simulink model "template_2018a"  (R2018a)
settings: Solver=ode45  StartTime=0.0  StopTime=0.75  MaxStep=1e-4  RelTol=1e-3  EnableMultiTasking=on
undefined symbols (not defined in the file or in its folder): KD, KI, KP
settings Model: Creator=Joe  LastModifiedBy=Adam Minnich
settings DataIOCC: LimitDataPoints=on  SaveFormat=Array
settings OptimizationCC: LifeSpan=inf
settings DebuggingCC: UnderspecifiedInitializationDetection=Classic  MergeDetectMultiDrivingBlocksExec=none  SolverPrmCheckMsg=warning  SFUnexpectedBacktrackingDiag=warning  SFNoUnconditionalDefaultTransitionDiag=warning  SFExecutionAtInitializationDiag=none
settings HardwareCC: ProdBitPerPointer=32  ProdBitPerSizeT=32  ProdBitPerPtrDiffT=32  ProdLargestAtomicFloat=None  ProdIntDivRoundTo=Undefined  ProdEndianess=Unspecified  ProdWordSize=32  ProdHWDeviceType=32-bit Generic
settings ModelReferenceCC: PropagateSignalLabelsOutOfModel=off
settings CodeAppCC: StateflowObjectComments=on
settings GRTTargetCC: TargetLangStandard=C89/C90 (ANSI)  GeneratePreprocessorConditionals=Disable all
settings ConfigComp: CovMetricSettings=dw  CovHtmlReporting=on  CovSaveCumulativeToWorkspaceVar=on  CovSaveSingleToWorkspaceVar=on  CovExternalEMLEnable=off  CovSFcnEnable=off

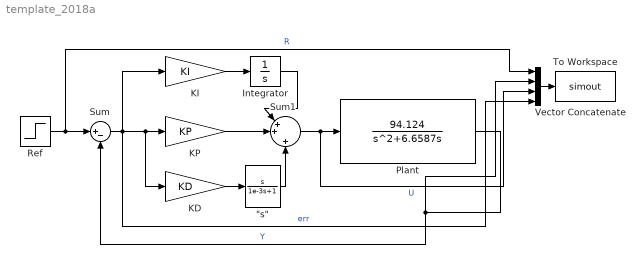
== system template_2018a ==
  "\"s\"" : TransferFcn  Numerator=[1 0]  Denominator=[1e-3 1]
  Integrator : Integrator
  KD : Gain  Gain=KD
  KI : Gain  Gain=KI
  KP : Gain  Gain=KP
  Plant : TransferFcn  Numerator=[94.124]  Denominator=[1 6.6587 0]
  Ref : Step  Time=0  After=pi/2  SampleTime=0
  Sum : Sum  Inputs=|+-
  Sum1 : Sum  Inputs=|++|+
  To Workspace : ToWorkspace  VariableName=simout  SaveFormat=Structure With Time  SampleTime=-1
  Vector Concatenate : Concatenate  NumInputs=4
  wires:
  Ref/1 -> Sum/1, Vector Concatenate/1  "R"
  Sum/1 -> KD/1, KP/1, KI/1, Vector Concatenate/4  "err"
  Plant/1 -> Vector Concatenate/2, Sum/2  "Y"
  Sum1/1 -> Vector Concatenate/3, Plant/1  "U"
  Vector Concatenate/1 -> To Workspace/1
  KP/1 -> Sum1/2
  KI/1 -> Integrator/1
  Integrator/1 -> Sum1/1
  KD/1 -> "\"s\""/1
  "\"s\""/1 -> Sum1/3
